simulink model "CoefMomentDamping_TestModel"  (R2014a)
settings: Solver=ode45  StartTime=0.0  StopTime=10.0  RelTol=1e-3
libraries: rocket_angular_flight_library x2
settings Model: Creator=scorpii  LastModifiedBy=scorpii

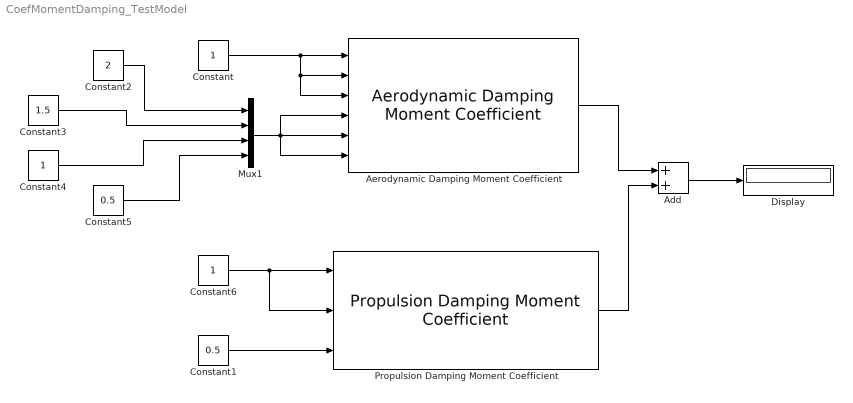
== system CoefMomentDamping_TestModel ==
  Add : Sum
  Aerodynamic Damping Moment Coefficient : rocket_angular_flight_library/Aerodynamic Damping Moment Coefficient
  Constant : Constant
  Constant1 : Constant  Value=0.5
  Constant2 : Constant  Value=2
  Constant3 : Constant  Value=1.5
  Constant4 : Constant
  Constant5 : Constant  Value=0.5
  Constant6 : Constant
  Display : Display
  Mux1 : Mux
  Propulsion Damping Moment Coefficient : rocket_angular_flight_library/Propulsion Damping Moment Coefficient
  wires:
  Aerodynamic Damping Moment Coefficient/1 -> Add/1
  Propulsion Damping Moment Coefficient/1 -> Add/2
  Add/1 -> Display/1
  Mux1/1 -> Aerodynamic Damping Moment Coefficient/4, Aerodynamic Damping Moment Coefficient/6, Aerodynamic Damping Moment Coefficient/5
  Constant2/1 -> Mux1/1
  Constant3/1 -> Mux1/2
  Constant4/1 -> Mux1/3
  Constant5/1 -> Mux1/4
  Constant/1 -> Aerodynamic Damping Moment Coefficient/3, Aerodynamic Damping Moment Coefficient/2, Aerodynamic Damping Moment Coefficient/1
  Constant6/1 -> Propulsion Damping Moment Coefficient/2, Propulsion Damping Moment Coefficient/1
  Constant1/1 -> Propulsion Damping Moment Coefficient/3
